simulink model "roll_ap"  (R2016a)
settings: Solver=FixedStepDiscrete  SolverMode=SingleTasking  StartTime=0.0  StopTime=25  FixedStep=1/40  RelTol=1e-3
model workspace (MAT data in the model file):
  dispGain = Simulink.Parameter
  dispGain.Value = 1
  dispGain.DataType = 'auto'
  dispGain.Dimensions = [1 1]
  hdgGain = Simulink.Parameter
  hdgGain.Value = 0.015
  hdgGain.DataType = 'auto'
  hdgGain.Min = 0
  hdgGain.Dimensions = [1 1]
  intGain = Simulink.Parameter
  intGain.Value = 1
  intGain.DataType = 'auto'
  intGain.Dimensions = [1 1]
  rateGain = Simulink.Parameter
  rateGain.Value = 3
  rateGain.DataType = 'auto'
  rateGain.Dimensions = [1 1]
undefined symbols (not defined in the file or in its folder): cmdLim, dispLim, intLim, rateLim
libraries: simulink x2
settings Model: RequirementInfo={} %GIDa_fe9045fd_0412_4b6e_8206_617cc20e6fde  ParameterArgumentNames=dispGain,intGain,rateGain,hdgGain  Creator=bpotter  LastModifiedBy=ceren.gebizli
settings DataIOCC: ExternalInput=apin  LoadExternalInput=on  SaveFormat=StructureWithTime  DSMLogging=off  OutputSaveName=Ail_Cmd  SignalLoggingName=roll_ap_logsout
settings OptimizationCC: BlockReduction=off  DefaultParameterBehavior=Inlined  InlineInvariantSignals=on  ExpressionDepthLimit=2147483647  EfficientFloat2IntCast=on  EfficientMapNaN2IntZero=off  OptimizeModelRefInitCode=on  MaxStackSize=inf
settings DebuggingCC: SignalInfNanChecking=error  SignalRangeChecking=error  ReadBeforeWriteMsg=EnableAllAsError  WriteAfterWriteMsg=EnableAllAsError  WriteAfterReadMsg=EnableAllAsError  AlgebraicLoopMsg=error  ArtificialAlgebraicLoopMsg=error  SaveWithDisabledLinksMsg=error  SaveWithParameterizedLinksMsg=error  CheckExecutionContextPreStartOutputMsg=on  CheckExecutionContextRuntimeOutputMsg=on  BlockPriorityViolationMsg=error  MaxConsecutiveZCsMsg=warning  SolverPrmCheckMsg=error  InheritedTsInSrcMsg=error  SingleTaskRateTransMsg=error  TasksWithSamePriorityMsg=error  SigSpecEnsureSampleTimeMsg=error  CheckMatrixSingularityMsg=error  IntegerOverflowMsg=error  ParameterUnderflowMsg=error  ParameterPrecisionLossMsg=error  ParameterTunabilityLossMsg=error  UnderSpecifiedDataTypeMsg=error  UnnecessaryDatatypeConvMsg=warning  VectorMatrixConversionMsg=error  SignalLabelMismatchMsg=error  UnconnectedInputMsg=error  UnconnectedOutputMsg=error  UnconnectedLineMsg=error  SFcnCompatibilityMsg=error  UniqueDataStoreMsg=error  BusObjectLabelMismatch=error  RootOutportRequireBusObject=error  AssertControl=DisableAll  ModelReferenceIOMsg=error  ModelReferenceIOMismatchMessage=error  UnknownTsInhSupMsg=error  ModelReferenceDataLoggingMessage=error  ModelReferenceExtraNoncontSigs=none  StateNameClashWarn=warning  StrictBusMsg=ErrorOnBusTreatedAsVector  NonBusSignalsTreatedAsBus=error  IntegerSaturationMsg=error
settings HardwareCC: ProdBitPerPointer=32  ProdLargestAtomicFloat=None  ProdEndianess=BigEndian  ProdWordSize=32  ProdHWDeviceType=32-bit Embedded Processor  TargetHWDeviceType=32-bit Generic
settings ModelReferenceCC: PropagateSignalLabelsOutOfModel=off
settings RTWCC: SystemTargetFile=ert.tlc  TemplateMakefile=ert_default_tmf  GenerateReport=on  RTWVerbose=off  IncludeHyperlinkInReport=on  LaunchReport=on  PortableWordSizes=on  GenerateTraceInfo=on  GenerateTraceReport=on  GenerateTraceReportSl=on  GenerateTraceReportSf=on  GenerateTraceReportEml=on
settings CodeAppCC: ForceParamTrailComments=on  IgnoreCustomStorageClasses=off  MaxIdLength=63  MangleLength=4  CustomSymbolStrType=$N$R$M  InternalIdentifier=Classic  ReqsInCode=on
settings ERTTargetCC: UtilityFuncGeneration=Shared location  IncludeMdlTerminateFcn=off  GeneratePreprocessorConditionals=Disable all  SuppressErrorStatus=on  SupportAbsoluteTime=off  SupportNonFinite=off  SupportComplex=off  ParenthesesLevel=Maximum  MultiInstanceErrorCode=None  ERTCustomFileTemplate=example_file_process.tlc  PreserveExpressionOrder=on  PreserveIfCondition=on  ConvertIfToSwitch=off  SuppressUnreachableDefaultCases=off
settings ConfigComp: CovSaveName=covdata_rollAP  CovMetricSettings=dcmtrzoiwe  CovHTMLOptions=-sRT=1 -aTS=1 -bRG=1 -bTC=1 -hTR=1 -nFC=0 -scm=1 -bcm=1 -xEv=0  CovHtmlReporting=off  CovSaveSingleToWorkspaceVar=off  CovCumulativeVarName=covCumulativeData_rollAP  CovCumulativeReport=on  CovReportOnPause=off  PSOpenProjectManager=on  PSSendToPolyspaceServer=on  PSModelRefVerifDepth=All  PSAutoStubLUT=off  DVMakeOutputFilesUnique=off  DVMaxTestCaseSteps=500  DVTestSuiteOptimization=CombinedObjectives (Nonlinear Extended)  DVDetectActiveLogic=on  DVSaveDataFile=off  DVSaveHarnessModel=on  DVModelReferenceHarness=on  DVSaveReport=on

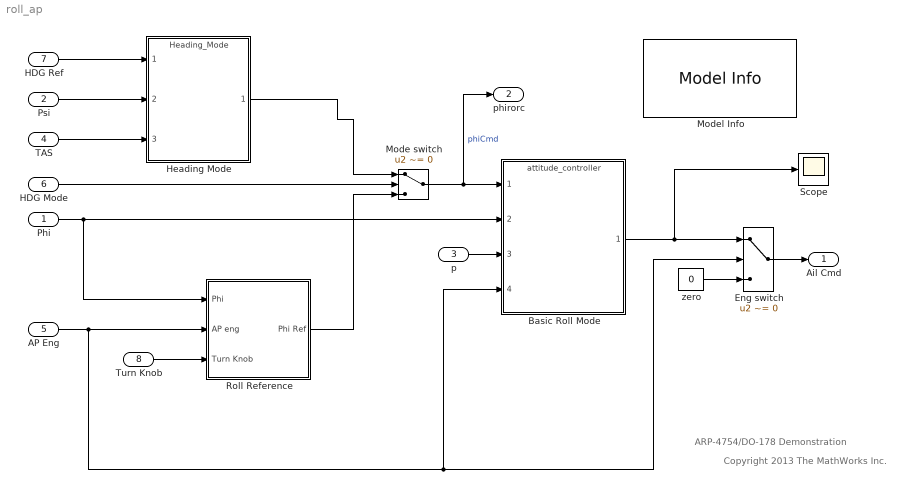
== system roll_ap ==
  note: Copyright 2013 The MathWorks Inc.
  note: ARP-4754/DO-178 Demonstration
  Phi : Inport  RequirementInfo={'other' 'do178b_autopilot_requirements.docx' '@Simulink_requirement_item_3' 'true' '1.3. Roll Hold Reference' ' ' ; 'other' 'do178b_autopilot_requirements.docx' '@Simulink_requirement_item_4' 'true' '1.4. Roll Performance' '' } %GIDa_040c2d73_6311_42f9_964f_56f1fff3d8d8  OutMin=-180  OutMax=180  OutDataTypeStr=double  PortDimensions=1  SampleTime=1/40  Interpolate=off
  Psi : Inport  RequirementInfo={'other' 'do178b_autopilot_requirements.docx' '@Simulink_requirement_item_10' 'true' '1.10. Heading Performance' '' } %GIDa_aa699f91_96f0_401b_acdb_f9b4b0743533  Port=2  OutMin=-180  OutMax=180  OutDataTypeStr=double  PortDimensions=1  SampleTime=1/40  Interpolate=off
  p : Inport  RequirementInfo={'other' 'do178b_autopilot_requirements.docx' '@Simulink_requirement_item_4' 'true' '1.4. Roll Performance' '' } %GIDa_91b6e343_cedd_4c09_9e82_9cc09e4312a7  Port=3  OutMin=-180  OutMax=180  OutDataTypeStr=double  PortDimensions=1  SampleTime=1/40  Interpolate=off
  TAS : Inport  RequirementInfo={'other' 'do178b_autopilot_requirements.docx' '@Simulink_requirement_item_10' 'true' '1.10. Heading Performance' '' } %GIDa_9daa2c3d_09c1_4ac6_a206_1425f5f778cd  Port=4  OutMin=0  OutMax=1000  OutDataTypeStr=double  PortDimensions=1  SampleTime=1/40  Interpolate=off
  AP Eng : Inport  RequirementInfo={'other' 'do178b_autopilot_requirements.docx' '@Simulink_requirement_item_1' 'true' '1.1. Roll Autopilot Engage Control' ' ' ; 'other' 'do178b_autopilot_requirements.docx' '@Simulink_requirement_item_3' 'true' '1.3. Roll Hold Reference' ' ' ; 'other' 'do178b_autopilot_requirements.docx' '@Simulink_requirement_item_4' 'true' '1.4. Roll Performance' '' } %GIDa_dbf8c750_871c_42fc_8ea1_57838e97fa97  Port=5  OutDataTypeStr=boolean  PortDimensions=1  SampleTime=1/40  Interpolate=off
  HDG Mode : Inport  RequirementInfo={'other' 'do178b_autopilot_requirements.docx' '@Simulink_requirement_item_2' 'true' '1.2. Roll Hold Mode' ' ' ; 'other' 'do178b_autopilot_requirements.docx' '@Simulink_requirement_item_8' 'true' '1.8. Heading Hold Mode' '' } %GIDa_3d1fd2be_b046_42ef_8f3c_1955bceadbb7  Port=6  OutDataTypeStr=boolean  PortDimensions=1  SampleTime=1/40  Interpolate=off
  HDG Ref : Inport  RequirementInfo={'other' 'do178b_autopilot_requirements.docx' '@Simulink_requirement_item_9' 'true' '1.9. Heading Hold Reference' ' ' ; 'other' 'do178b_autopilot_requirements.docx' '@Simulink_requirement_item_10' 'true' '1.10. Heading Performance' '' } %GIDa_96162cda_cb1a_490e_8dac_f861526aad50  Port=7  OutMin=-180  OutMax=180  OutDataTypeStr=double  PortDimensions=1  SampleTime=1/40  Interpolate=off
  Turn Knob : Inport  RequirementInfo={'other' 'do178b_autopilot_requirements.docx' '@Simulink_requirement_item_3' 'true' '1.3. Roll Hold Reference' '' } %GIDa_fa976ccd_1ea9_4823_b673_fef2768ad601  Port=8  OutMin=-45  OutMax=45  OutDataTypeStr=double  PortDimensions=1  SampleTime=1/40  Interpolate=off
  Basic Roll Mode : ModelReference  RequirementInfo={'other' 'do178b_autopilot_requirements.docx' '@Simulink_requirement_item_4' 'true' '1.4. Roll Performance' '' ; 'other' 'do178b_autopilot_requirements.docx' '@Simulink_requirement_item_5' 'true' '1.5. Roll Rate Limit' '' ; 'other' 'do178b_autopilot_requirements.docx' '@Simulink_requirement_item_6' 'true' '1.6. Roll Angle Limit' '' ; 'other' 'do178b_autopilot_requirements.docx' '@Simulink_requirement_item_7' 'true' '1.7. Aileron Angle Limit' '' } %GIDa_94fed7b0_f432_43f5_a2d9_2abccf075f5b  ModelNameDialog=attitude_controller  ParameterArgumentNames=dispGain,dispLim,rateGain,rateLim,intGain,intLim,cmdLim  ParameterArgumentValues=dispGain,30,rateGain,6,intGain,5,15  SimulationMode=Normal  ModelReferenceVersion=1.67
  Eng switch : Switch  RequirementInfo={'other' 'do178b_autopilot_requirements.docx' '' 'true' '1.1. Roll Autopilot Engage Control' ' ' } %GIDa_1f89e2a1_f10b_411b_80f1_4c7070559f04  Criteria=u2 ~= 0
  Heading Mode : ModelReference  RequirementInfo={'other' 'do178b_autopilot_requirements.docx' '@Simulink_requirement_item_10' 'true' '1.10. Heading Performance' '' } %GIDa_e0954c89_e814_46d2_8f67_6d4b1cdfab81  ModelNameDialog=Heading_Mode  ParameterArgumentNames=hdgGain  ParameterArgumentValues=hdgGain  SimulationMode=Normal  ModelReferenceVersion=1.147
  Mode switch : Switch  RequirementInfo={'other' 'do178b_autopilot_requirements.docx' '@Simulink_requirement_item_2' 'true' '1.2. Roll Hold Mode' ' ' ; 'other' 'do178b_autopilot_requirements.docx' '@Simulink_requirement_item_4' 'true' '1.4. Roll Performance' ' ' ; 'other' 'do178b_autopilot_requirements.docx' '@Simulink_requirement_item_8' 'true' '1.8. Heading Hold Mode' ' ' ; 'other' 'do178b_autopilot_requirements.docx' '@Simulink_requirement_item_10' 'true' '1.10. Heading Performance' '' } %GIDa_89518de0_411a_4ee8_869d_c7ed5e5087e3  Criteria=u2 ~= 0
  Model Info : simulink/Model-Wide Utilities/Model Info  RequirementInfo={} %GIDa_ca11a4b2_f22f_461f_8532_eb2c7aa53101  InitialSaveTempField=(Not available in SLX model file format)#|#(Not available in SLX model file format)#|#(Not available in SLX model file format)#|#(Not available in SLX model file format)#|#(Not available in SLX model file format)#|#(Not available in SLX model file format)#|#(Not available in SLX model file format)#|#(Not available in SLX model file format)#|#(Not available in SLX model file format)#|#  InitialBlockCM=Microsoft Visual SourceSafe  BlockCM=Microsoft Visual SourceSafe  Frame=on  SaveTempField=(Not available in SLX model file format)#|#(Not available in SLX model file format)#|#(Not available in SLX model file format)#|#(Not available in SLX model file format)#|#(Not available in SLX model file format)#|#(Not available in SLX model file format)#|#(Not available in SLX model file format)#|#(Not available in SLX model file format)#|#(Not available in SLX model file format)#|#  DisplayStringWithTags=|  HorizontalTextAlignment=Left  LeftAlignmentValue=0.02  SourceBlockDiagram=roll_ap  TagMaxNumber=20  CMTag1=$Author: $  CMTag2=$Date: $  CMTag3=$Revision: $  CMTag4=$Archive: $  CMTag5=$Header: $  CMTag6=$Logfile: $  CMTag7=$Modtime: $  CMTag8=$Workfile: $  CMTag9=$JustDate: $
      | Roll Autopilot
      | Author: %<LastModifiedBy>
      | Model Version: %<ModelVersion>
      | Date: %<LastModificationDate>
  Roll Reference : Subsystem  RequirementInfo={'other' 'do178b_autopilot_requirements.docx' '@Simulink_requirement_item_3' 'true' '1.3. Roll Hold Reference' '' } %GIDa_c8cf196e_df7c_4434_8b0c_5575b514a7cf  TreatAsAtomicUnit=on
      settings: RTWSystemCode=Inline
  Scope : Scope
  zero : Constant  RequirementInfo={'other' 'do178b_autopilot_requirements.docx' '' 'true' '1.1. Roll Autopilot Engage Control' '' } %GIDa_8c99e557_6257_4659_beae_770a67a6ac3a  Value=0  OutDataTypeStr=double
  Ail Cmd : Outport  RequirementInfo={'other' 'do178b_autopilot_requirements.docx' '' 'true' '1.1. Roll Autopilot Engage Control' ' ' } %GIDa_02b61f6d_71d4_4b0d_89ac_bfbca808eb5f  OutDataTypeStr=double  PortDimensions=1  SampleTime=1/40
  " phirorc" : Outport  RequirementInfo={'other' 'do178b_autopilot_requirements.docx' '' 'true' '1.1. Roll Autopilot Engage Control' ' ' } %GIDa_c4b6b638_aed5_4cc5_9198_730f18106828  Port=2  OutDataTypeStr=double  PortDimensions=1  SampleTime=1/40
  wires:
  HDG Ref/1 -> Heading Mode/1
  Phi/1 -> Roll Reference/1(Phi), Basic Roll Mode/2
  p/1 -> Basic Roll Mode/3
  Psi/1 -> Heading Mode/2
  TAS/1 -> Heading Mode/3
  Mode switch/1 -> " phirorc"/1, Basic Roll Mode/1  "phiCmd"
  HDG Mode/1 -> Mode switch/2
  Heading Mode/1 -> Mode switch/1
  AP Eng/1 -> Eng switch/2, Basic Roll Mode/4, Roll Reference/2(AP eng)
  Basic Roll Mode/1 -> Scope/1, Eng switch/1
  Eng switch/1 -> Ail Cmd/1
  zero/1 -> Eng switch/3
  Roll Reference/1(Phi Ref) -> Mode switch/3
  Turn Knob/1 -> Roll Reference/3(Turn Knob)

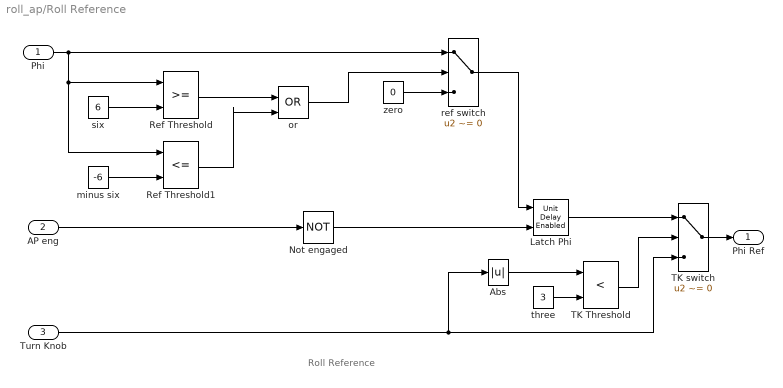
== system roll_ap/Roll Reference ==
  note: Roll Reference
  Phi : Inport  RequirementInfo={'other' 'do178b_autopilot_requirements.docx' '@Simulink_requirement_item_3' 'true' '1.3. Roll Hold Reference' '' } %GIDa_365246ee_5fe4_4d20_a97b_c1028127f0f0
  AP eng : Inport  RequirementInfo={'other' 'do178b_autopilot_requirements.docx' '@Simulink_requirement_item_3' 'true' '1.3. Roll Hold Reference' '' } %GIDa_d4efac82_9df2_4cb3_8b82_71e18ecb0348  Port=2
  Turn Knob : Inport  RequirementInfo={'other' 'do178b_autopilot_requirements.docx' '@Simulink_requirement_item_3' 'true' '1.3. Roll Hold Reference' '' } %GIDa_d8bc0518_f9fa_4c47_a645_e8b5f2762f20  Port=3
  Abs : Abs  RequirementInfo={'other' 'do178b_autopilot_requirements.docx' '@Simulink_requirement_item_3' 'true' '1.3. Roll Hold Reference' '' } %GIDa_c8abfe5d_55a5_4c1b_9135_acd6c20e2232
  Latch Phi : simulink/Additional Math & Discrete/Additional Discrete/Unit Delay Enabled  RequirementInfo={'other' 'do178b_autopilot_requirements.docx' '@Simulink_requirement_item_3' 'true' '1.3. Roll Hold Reference' '' } %GIDa_8c2a6474_62f7_4673_9b80_815aaee792d7  vinit=0.0  tsamp=1/40
  Not engaged : Logic  RequirementInfo={'other' 'do178b_autopilot_requirements.docx' '@Simulink_requirement_item_3' 'true' '1.3. Roll Hold Reference' '' } %GIDa_e52c6893_d81b_4f15_89c3_12b6a83c27b2  Operator=NOT  IconShape=distinctive  AllPortsSameDT=off  OutDataTypeStr=boolean
  Ref Threshold : RelationalOperator  RequirementInfo={'other' 'do178b_autopilot_requirements.docx' '@Simulink_requirement_item_3' 'true' '1.3. Roll Hold Reference' '' } %GIDa_be19764a_4253_499a_816c_5a218f85ba52  OutDataTypeStr=boolean  InputSameDT=on
  Ref Threshold1 : RelationalOperator  RequirementInfo={'other' 'do178b_autopilot_requirements.docx' '@Simulink_requirement_item_3' 'true' '1.3. Roll Hold Reference' '' } %GIDa_66db49a9_aa40_43ab_9d6f_efe68ac443ed  Operator=<=  OutDataTypeStr=boolean  InputSameDT=on
  TK Threshold : RelationalOperator  RequirementInfo={'other' 'do178b_autopilot_requirements.docx' '@Simulink_requirement_item_3' 'true' '1.3. Roll Hold Reference' '' } %GIDa_9859b478_272f_4974_a36c_6c4f8c030643  Operator=<  OutDataTypeStr=boolean  InputSameDT=on
  TK switch : Switch  RequirementInfo={'other' 'do178b_autopilot_requirements.docx' '@Simulink_requirement_item_3' 'true' '1.3. Roll Hold Reference' '' } %GIDa_804165d0_89eb_4919_a8d1_f2310004f7d9  Criteria=u2 ~= 0
  minus six : Constant  RequirementInfo={'other' 'do178b_autopilot_requirements.docx' '@Simulink_requirement_item_3' 'true' '1.3. Roll Hold Reference' '' } %GIDa_3d290e71_7846_48ec_bba2_120ec195a4d2  Value=-6
  or : Logic  RequirementInfo={'other' 'do178b_autopilot_requirements.docx' '@Simulink_requirement_item_3' 'true' '1.3. Roll Hold Reference' '' } %GIDa_6038a0c7_77ff_4867_84b3_3e7893f58df6  Operator=OR  IconShape=distinctive  OutDataTypeStr=boolean
  ref switch : Switch  RequirementInfo={'other' 'do178b_autopilot_requirements.docx' '@Simulink_requirement_item_3' 'true' '1.3. Roll Hold Reference' '' } %GIDa_a4746381_6ebe_4e3d_83b9_b49d14a3af5e  Criteria=u2 ~= 0
  six : Constant  RequirementInfo={'other' 'do178b_autopilot_requirements.docx' '@Simulink_requirement_item_3' 'true' '1.3. Roll Hold Reference' '' } %GIDa_0870d8d6_d29f_4cb4_9c0c_9079ccdb7173  Value=6
  three : Constant  RequirementInfo={'other' 'do178b_autopilot_requirements.docx' '@Simulink_requirement_item_3' 'true' '1.3. Roll Hold Reference' '' } %GIDa_6228e2c4_8022_4eaf_90d6_7c47f19fb0a2  Value=3  OutDataTypeStr=double
  zero : Constant  RequirementInfo={'other' 'do178b_autopilot_requirements.docx' '@Simulink_requirement_item_3' 'true' '1.3. Roll Hold Reference' '' } %GIDa_e4775650_e5c7_4c74_aef4_71c144af3cbc  Value=0
  Phi Ref : Outport  RequirementInfo={'other' 'do178b_autopilot_requirements.docx' '@Simulink_requirement_item_3' 'true' '1.3. Roll Hold Reference' '' } %GIDa_75cfa841_d3b7_422f_bd46_8ed4a58fc723
  wires:
  Not engaged/1 -> Latch Phi/2
  ref switch/1 -> Latch Phi/1
  Latch Phi/1 -> TK switch/1
  TK Threshold/1 -> TK switch/2
  Turn Knob/1 -> TK switch/3, Abs/1
  three/1 -> TK Threshold/2
  Abs/1 -> TK Threshold/1
  Phi/1 -> ref switch/1, Ref Threshold/1, Ref Threshold1/1
  AP eng/1 -> Not engaged/1
  TK switch/1 -> Phi Ref/1
  six/1 -> Ref Threshold/2
  zero/1 -> ref switch/3
  or/1 -> ref switch/2
  Ref Threshold/1 -> or/1
  Ref Threshold1/1 -> or/2
  minus six/1 -> Ref Threshold1/2
